simulink model "konstv"  (R2014b)
settings: Solver=ode45  StartTime=0.0  StopTime=10.0  RelTol=1e-3
settings Model: Creator=sigurd  LastModifiedBy=sigurd

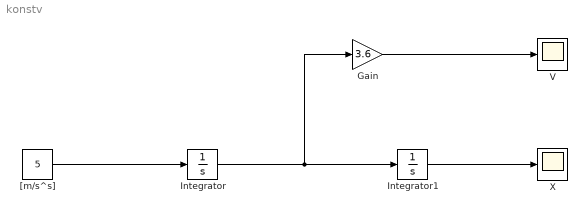
== system konstv ==
  Gain : Gain  Gain=3.6
  Integrator : Integrator  InitialCondition=50/3.6
  Integrator1 : Integrator
  V : Scope
  X : Scope
  "[m/s^s]" : Constant  Value=5
  wires:
  Gain/1 -> V/1
  "[m/s^s]"/1 -> Integrator/1
  Integrator/1 -> Gain/1, Integrator1/1
  Integrator1/1 -> X/1
